simulink model "tirePressureMonitoringSystem"  (R2022a)
settings: configuration reference "CommonConfigurationSet" (kept outside this file)
model workspace (MATLAB code in the model file + MAT data in the model file):
  cmdLim = Simulink.Parameter
  cmdLim.Value = 15
  cmdLim.Description = 'Limit for controlling the maximum surface command angle.'
  cmdLim.Min = 0
  cmdLim.Max = 90
  cmdLim.DocUnits = 'deg'
  dispGain = Simulink.Parameter
  dispGain.Value = 0.75
  dispGain.Description = 'Gain applied to the displacement error.'
  dispGain.Min = 0
  dispGain.Max = []
  dispGain.DocUnits = 'deg/sec/deg'
  dispLim = Simulink.Parameter
  dispLim.Value = 30
  dispLim.Description = 'Limit for controlling the maximum commanded angle.'
  dispLim.Min = 0
  dispLim.Max = 180
  dispLim.DocUnits = 'deg'
  intGain = Simulink.Parameter
  intGain.Value = 0.5
  intGain.Description = 'Gain applied to the integral error.'
  intGain.Min = 0
  intGain.Max = []
  intGain.DocUnits = 'deg/sec/deg/sec'
  intLim = Simulink.Parameter
  intLim.Value = 5
  intLim.Description = 'Limit for controlling the maximum commanded angle.'
  intLim.Min = 0
  intLim.Max = 90
  intLim.DocUnits = 'deg'
  rateGain = Simulink.Parameter
  rateGain.Value = 2
  rateGain.Description = 'Gain applied to the rate error.'
  rateGain.Min = 0
  rateGain.Max = []
  rateGain.DocUnits = 'deg/deg/sec'
  rateLim = Simulink.Parameter
  rateLim.Value = 6
  rateLim.Description = 'Limit for controlling the maximum commanded angle.'
  rateLim.Min = 0
  rateLim.Max = 180
  rateLim.DocUnits = 'deg/sec'
  hdgGain = Simulink.Parameter
  hdgGain.Value = 0.015
  CONTROLLER_CLIENT_ID_LIST = Simulink.Parameter
  CONTROLLER_CLIENT_ID_LIST.Value(1).device_id = [1; 1; 1; 1; 1; 1; 1; 1; 1; 1]
  CONTROLLER_CLIENT_ID_LIST.Value(2).device_id = [2; 2; 2; 2; 2; 2; 2; 2; 2; 2]
  CONTROLLER_CLIENT_ID_LIST.Value(3).device_id = [3; 3; 3; 3; 3; 3; 3; 3; 3; 3]
  CONTROLLER_CLIENT_ID_LIST.Value(4).device_id = [4; 4; 4; 4; 4; 4; 4; 4; 4; 4]
  CONTROLLER_CLIENT_ID_LIST.Description = '[ initializedDeviceIDBusTypeConstructor( repmat( 1, 10, 1 ) ); initializedDeviceIDBusTypeConstructor( repmat( 2, 10, 1 ) ); initializedDeviceIDBusTypeConstructor( repmat( 3, 10, 1 ) ); initializedDeviceIDBusTypeConstructor( repmat( 4, 10, 1 ) ) ] '
  CONTROLLER_CLIENT_ID_LIST.DataType = 'struct'
  CONTROLLER_CLIENT_ID_LIST.Complexity = 'real'
  CONTROLLER_CLIENT_ID_LIST.Dimensions = [4 1]
  UNRELATED_DEVICE_ID = Simulink.Parameter
  UNRELATED_DEVICE_ID.Value.device_id = [5; 5; 5; 5; 5; 5; 5; 5; 5; 5]
  UNRELATED_DEVICE_ID.Description = 'SensorTargetSpecificCodeExternalDependency.initializedDeviceIDBusTypeConstructor( repmat( uint8( 5 ), 10, 1 ) )'
  UNRELATED_DEVICE_ID.DataType = 'struct'
  UNRELATED_DEVICE_ID.Complexity = 'real'
  UNRELATED_DEVICE_ID.Dimensions = [1 1]
undefined symbols (not defined in the file): m, SENSOR_SAMPLE_TIME
settings Model: RequirementInfo={} %GIDa_fe9045fd_0412_4b6e_8206_617cc20e6fde  DataDictionary=systemData.sldd  EnableAccessToBaseWorkspace=off  FPTRunName=Active  Creator=The MathWorks, Inc.  LastModifiedBy=The MathWorks, Inc.
settings ConfigSetRef: SourceName=CommonConfigurationSet

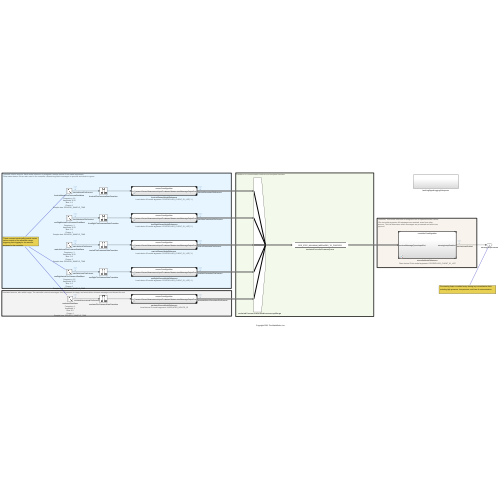
[thumbnail: Simulink's stored preview of the top-level diagram]
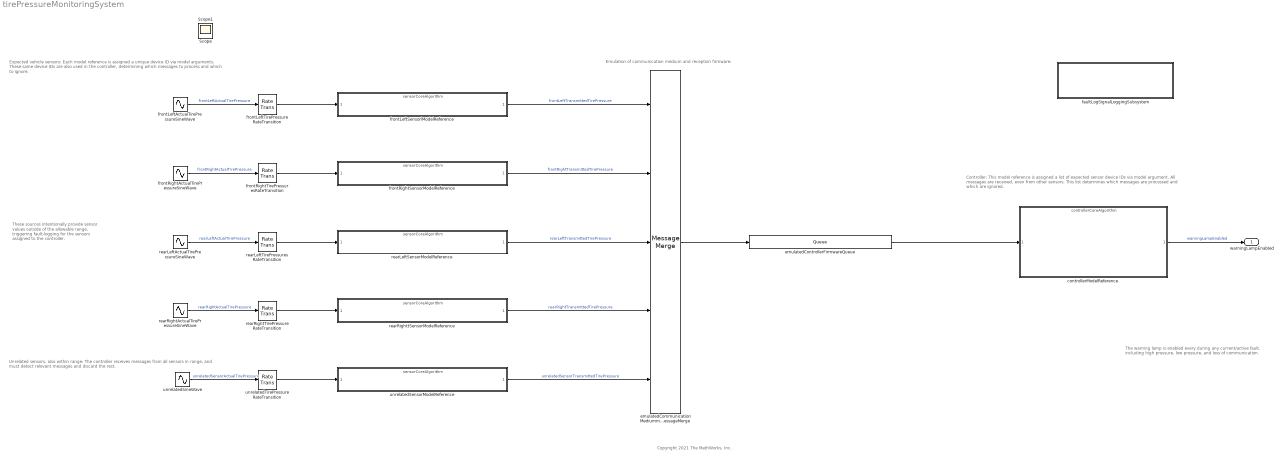
== system tirePressureMonitoringSystem ==
  note: Emulation of communication medium and reception firmware:
  note: Controller: This model reference is assigned a list of expected sensor device
      |  IDs via model argument. All messages are received, even from other
      | sensors. This list determines which messages are processed and which are
      |  ignored.
  note: Unrelated sensors, also within range: The controller receives messages from all sensors in range, and must detect relevant messages and discard the rest.
  note: Expected vehicle sensors: Each model reference is assigned a unique device ID via model arguments.
      | These same device IDs are also used in the controller, determining which messages to process and which to ignore.
  note: The warning lamp is enabled every during any current/active fault, including high pressure, low pressure, and loss of communication.
  note: These sources intentionally provide sensor values outside of the allowable range, triggering fault-logging for the sensors assigned to the controller.
  note: Copyright 2021 The MathWorks, Inc.
  controllerModelReference : ModelReference  InputPortMessageModes=m  ModelNameDialog=controllerCoreAlgorithm  UsingDefaultArgumentValue=0  SimulationMode=Normal  ModelReferenceVersion=4.0
      settings: AttributesFormatString=Client device ID list model argument: %<ParameterArgumentValuesAsString>
  emulatedCommunicationMediummessageMerge : MessageMerge  InputPortMessageModes=m,m,m,m,m  OutputPortMessageModes=m  NumberInputPorts=5
      settings: InputPortMap=u1,u2,u3,u4,u5
  emulatedControllerFirmwareQueue : Queue  InputPortMessageModes=m  OutputPortMessageModes=m  OverwriteOldest=on  Capacity=PER_STEP_MAXIMUM_MESSAGES_TO_PROCESS  QueueType=LIFO
  faultLogSignalLoggingSubsystem : Subsystem
  frontLeftActualTirePressureSineWave : Sin  Amplitude=0.25  Bias=1.5  Frequency=0.5  SampleTime=SENSOR_SAMPLE_TIME
      settings: AttributesFormatString=|
      | Frequency: %<Frequency>
      | Amplitude: %<Amplitude>
      | Bias: %<Bias>
      | Phase: %<Phase>
      | Sample time: %<SampleTime>
  frontLeftSensorlModelReference : ModelReference  OutputPortMessageModes=m  ModelNameDialog=sensorCoreAlgorithm  UsingDefaultArgumentValue=0  ModelReferenceVersion=4.0
      settings: AttributesFormatString=Local device ID model argument: %<ParameterArgumentValuesAsString>
  frontLeftTirePressureRateTransition : RateTransition
  frontRightActualTirePressureSineWave : Sin  Amplitude=0.25  Bias=2.5  Phase=1  SampleTime=SENSOR_SAMPLE_TIME
      settings: AttributesFormatString=|
      | Frequency: %<Frequency>
      | Amplitude: %<Amplitude>
      | Bias: %<Bias>
      | Phase: %<Phase>
      | Sample time: %<SampleTime>
  frontRightSensorModelReference : ModelReference  OutputPortMessageModes=m  ModelNameDialog=sensorCoreAlgorithm  UsingDefaultArgumentValue=0  ModelReferenceVersion=4.0
      settings: AttributesFormatString=Local device ID model argument: %<ParameterArgumentValuesAsString>
  frontRightTirePressuresRateTransition : RateTransition
  rearLeftActualTirePressureSineWave : Sin  Amplitude=0.25  Bias=3.5  Phase=2  SampleTime=SENSOR_SAMPLE_TIME
      settings: AttributesFormatString=|
      | Frequency: %<Frequency>
      | Amplitude: %<Amplitude>
      | Bias: %<Bias>
      | Phase: %<Phase>
      | Sample time: %<SampleTime>
  rearLeftSensorModelReference : ModelReference  OutputPortMessageModes=m  ModelNameDialog=sensorCoreAlgorithm  UsingDefaultArgumentValue=0  ModelReferenceVersion=4.0
      settings: AttributesFormatString=Local device ID model argument: %<ParameterArgumentValuesAsString>
  rearLeftTirePressuresRateTransition : RateTransition
  rearRightActualTirePressureSineWave : Sin  Amplitude=0.25  Bias=4.5  Frequency=0.5  SampleTime=SENSOR_SAMPLE_TIME
      settings: AttributesFormatString=|
      | Frequency: %<Frequency>
      | Amplitude: %<Amplitude>
      | Bias: %<Bias>
      | Phase: %<Phase>
      | Sample time: %<SampleTime>
  rearRightTirePressureRateTransition : RateTransition
  rearRighttSensorModelReference : ModelReference  OutputPortMessageModes=m  ModelNameDialog=sensorCoreAlgorithm  UsingDefaultArgumentValue=0  ModelReferenceVersion=4.0
      settings: AttributesFormatString=Local device ID model argument: %<ParameterArgumentValuesAsString>
  unrelatedSensorModelReference : ModelReference  OutputPortMessageModes=m  ModelNameDialog=sensorCoreAlgorithm  UsingDefaultArgumentValue=0  ModelReferenceVersion=4.0
      settings: AttributesFormatString=Local device ID model argument: %<ParameterArgumentValuesAsString>
  unrelatedSineWave : Sin  Bias=5.5  Phase=4  SampleTime=SENSOR_SAMPLE_TIME
      settings: AttributesFormatString=|
      | Frequency: %<Frequency>
      | Amplitude: %<Amplitude>
      | Bias: %<Bias>
      | Phase: %<Phase>
      | Sample time: %<SampleTime>
  unrelatedTirePressureRateTransition : RateTransition
  warningLampEnabled : Outport
  Scope : Scope
  Scope1 : Scope
  wires:
  controllerModelReference/1 -> warningLampEnabled/1  "warningLampEnabled"
  unrelatedTirePressureRateTransition/1 -> unrelatedSensorModelReference/1
  unrelatedSineWave/1 -> unrelatedTirePressureRateTransition/1  "unrelatedSensorActualTirePressure"
  emulatedCommunicationMediummessageMerge/1 -> emulatedControllerFirmwareQueue/1
  frontLeftActualTirePressureSineWave/1 -> frontLeftTirePressureRateTransition/1  "frontLeftActualTirePressure"
  frontRightActualTirePressureSineWave/1 -> frontRightTirePressuresRateTransition/1  "frontRightActualTirePressure"
  rearRightActualTirePressureSineWave/1 -> rearRightTirePressureRateTransition/1  "rearRightActualTirePressure"
  frontLeftSensorlModelReference/1 -> emulatedCommunicationMediummessageMerge/1  "frontLeftTransmittedTirePressure"
  frontRightSensorModelReference/1 -> emulatedCommunicationMediummessageMerge/2  "frontRightTransmittedTirePressure"
  rearLeftSensorModelReference/1 -> emulatedCommunicationMediummessageMerge/3  "rearLeftTransmittedTirePressure"
  rearRighttSensorModelReference/1 -> emulatedCommunicationMediummessageMerge/4  "rearRightTransmittedTirePressure"
  frontLeftTirePressureRateTransition/1 -> frontLeftSensorlModelReference/1
  frontRightTirePressuresRateTransition/1 -> frontRightSensorModelReference/1
  rearLeftTirePressuresRateTransition/1 -> rearLeftSensorModelReference/1
  rearRightTirePressureRateTransition/1 -> rearRighttSensorModelReference/1
  emulatedControllerFirmwareQueue/1 -> controllerModelReference/1
  unrelatedSensorModelReference/1 -> emulatedCommunicationMediummessageMerge/5  "unrelatedSensorTransmittedTirePressure"
  rearLeftActualTirePressureSineWave/1 -> rearLeftTirePressuresRateTransition/1  "rearLeftActualTirePressure"

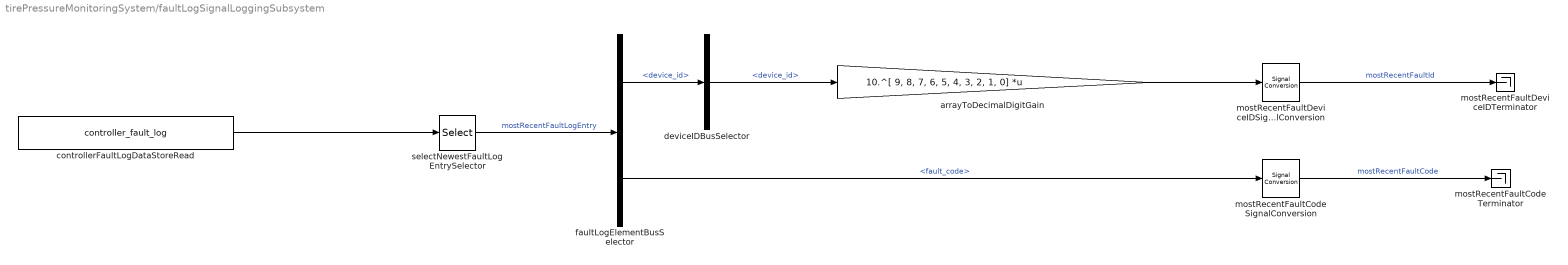
== system tirePressureMonitoringSystem/faultLogSignalLoggingSubsystem ==
  arrayToDecimalDigitGain : Gain  Gain=10.^[ 9, 8, 7, 6, 5, 4, 3, 2, 1, 0]  Multiplication=Matrix(K*u)
      settings: AttributesFormatString=Multiplication type: %<Multiplication>
  controllerFaultLogDataStoreRead : DataStoreRead  DataStoreName=controller_fault_log  IndexOptions=Index vector (dialog)  Indices=1  OutputSizes=1
  deviceIDBusSelector : BusSelector  OutputSignals=device_id
  faultLogElementBusSelector : BusSelector  OutputSignals=device_id,fault_code
  mostRecentFaultCodeSignalConversion : SignalConversion  OverrideOpt=off
  mostRecentFaultCodeTerminator : Terminator
  mostRecentFaultDeviceIDSignalConversion : SignalConversion  OverrideOpt=off
  mostRecentFaultDeviceIDTerminator : Terminator
  selectNewestFaultLogEntrySelector : Selector  IndexMode=Zero-based  InputPortWidth=10  IndexOptions=Index vector (dialog)  Indices=0  OutputSizes=1
  wires:
  controllerFaultLogDataStoreRead/1 -> selectNewestFaultLogEntrySelector/1
  deviceIDBusSelector/1 -> arrayToDecimalDigitGain/1  "<device_id>"
  faultLogElementBusSelector/2 -> mostRecentFaultCodeSignalConversion/1  "<fault_code>"
  mostRecentFaultDeviceIDSignalConversion/1 -> mostRecentFaultDeviceIDTerminator/1  "mostRecentFaultId"
  selectNewestFaultLogEntrySelector/1 -> faultLogElementBusSelector/1  "mostRecentFaultLogEntry"
  faultLogElementBusSelector/1 -> deviceIDBusSelector/1  "<device_id>"
  arrayToDecimalDigitGain/1 -> mostRecentFaultDeviceIDSignalConversion/1
  mostRecentFaultCodeSignalConversion/1 -> mostRecentFaultCodeTerminator/1  "mostRecentFaultCode"
